simulink model "CarE_Model"  (R2019b)
settings: Solver=VariableStepAuto  StartTime=0.0  StopTime=inf  RelTol=1e-3
(part 3 of 5)

== matlab function CarE_Model/CarE_System/Mapping Module/MATLAB Function to map intensity values to facial expressions ==
  data: contribution input; anger_val output; index input; disgust_val output; fear_val output; happiness_val output; neutral_val output; sadness_val output; surprise_val output; sum output; health_factor input
function [anger_val, disgust_val, fear_val, happiness_val, neutral_val, sadness_val, surprise_val, sum] = mapping(contribution, index, health_factor)
% % we see the heaviest weightage emotion
% % we calculate face expression values for that
% % then we move to second weightage emotion
% % calculate the face expression values for that
% % so on

% health factor(hf)decides the intensity of emotion
% % FINDING NORMALIZED HF VALUE
hf = (health_factor - 3)/5;

%% INITIALIZING THE VALUES
angerexp = zeros(22,1);
disgustexp = zeros(22,1);
fearexp = zeros(22,1);
happinessexp = zeros(22,1);
neutralexp = zeros(22,1);
sadnessexp = zeros(22,1);
surpriseexp = zeros(22,1);

intensity = zeros(22,1);
%checkvalout = zeros(7,1);

% For emotion on index value 1
exp1 = index(1);
switch(exp1)
    case 1
        % joy
        happinessexp(1) = 100;
        surpriseexp(1) = 0;
        intensity(1) = 100;
    case 2 
        % distress
        sadnessexp(1) = 100;
        angerexp(1) = 0;
        intensity(1) = 100;
    case 3
        % hope
        happinessexp(1) = 100;
        surpriseexp(1) = 0;
        intensity(1) = 20;
    case 4
        % fear
        fearexp(1) = 50;
        sadnessexp(1) = 50;
        intensity(1) = 20;
    case 5
        % satisfaction
        happinessexp(1) = 100;
        surpriseexp(1) = 0;
        intensity(1) = 80;
    case 6
        % fear_confirmed
        fearexp(1) = 50;
        sadnessexp(1) = 50;
        intensity(1) = 80;
    case 7
        % relief
        happinessexp(1) = 70;
        surpriseexp(1) = 30;
        intensity(1) = 700;
    case 8
        % disappointment
        fearexp(1) = 50;
        sadnessexp(1) = 50;
        intensity(1) = 80;
    case 9
        % happy_for
        happinessexp(1) = 100;
        surpriseexp(1) = 0;
        intensity(1) = 100;
    case 10
        % sorry_for
        fearexp(1) = 50;
        sadnessexp(1) = 50;
        intensity(1) = 100;
    case 11
        % gloating
        disgustexp(1) = 50;
        happinessexp(1) = 50;
        intensity(1) = 100;
    case 12
        % resentment
        angerexp(1) = 50;
        disgustexp(1) = 50;
        intensity(1) = 100;
    case 13
        % pride
        happinessexp(1) = 100;
        surpriseexp(1) = 0;
        intensity(1) = 100;
    case 14
        % shame
        sadnessexp(1) = 50;
        angerexp(1) = 50;
        intensity(1) = 100;
    case 15
        % admiration
        happinessexp(1) = 50;
        surpriseexp(1) = 50;
        intensity(1) = 100;
    case 16
        % reproach
        angerexp(1) = 50;
        disgustexp(1) = 50;
        intensity(1) = 100;
    case 17
        % gratitude
        happinessexp(1) = 100;
        surpriseexp(1) = 0;
        intensity(1) = 100;
    case 18
        % anger
        angerexp(1) = 100;
        disgustexp(1) = 0;
        intensity(1) = 100;
    case 19
        % gratification
        happinessexp(1) = 100;
        surpriseexp(1) = 0;
        intensity(1) = 100;
    case 20
        % remorse
        sadnessexp(1) = 100;
        angerexp(1) = 0;
        intensity(1) = 100;
    case 21
        % liking
        happinessexp(1) = 70;
        surpriseexp(1) = 30;
        intensity(1) = 100;
    case 22
        % disliking
        disgustexp(1) = 100;
        happinessexp(1) = 0;
        intensity(1) = 100;
    otherwise
        neutralexp(1) = 100;
        intensity(1) = 100;
end

% For emotion on index value 2
exp2 = index(2);
switch(exp2)
    case 1
        % joy
        happinessexp(2) = 100;
        surpriseexp(2) = 0;
        intensity(2) = 100;
    case 2 
        % distress
        sadnessexp(2) = 100;
        angerexp(2) = 0;
        intensity(2) = 100;
    case 3
        % hope
        happinessexp(2) = 100;
        surpriseexp(2) = 0;
        intensity(2) = 20;
    case 4
        % fear
        fearexp(2) = 50;
        sadnessexp(2) = 50;
        intensity(2) = 20;
    case 5
        % satisfaction
        happinessexp(2) = 100;
        surpriseexp(2) = 0;
        intensity(2) = 80;
    case 6
        % fear_confirmed
        fearexp(2) = 50;
        sadnessexp(2) = 50;
        intensity(2) = 80;
    case 7
        % relief
        happinessexp(2) = 70;
        surpriseexp(2) = 30;
        intensity(2) = 700;
    case 8
        % disappointment
        fearexp(2) = 50;
        sadnessexp(2) = 50;
        intensity(2) = 80;
    case 9
        % happy_for
        happinessexp(2) = 100;
        surpriseexp(2) = 0;
        intensity(2) = 100;
    case 10
        % sorry_for
        fearexp(2) = 50;
        sadnessexp(2) = 50;
        intensity(2) = 100;
    case 11
        % gloating
        disgustexp(2) = 50;
        happinessexp(2) = 50;
        intensity(2) = 100;
    case 12
        % resentment
        angerexp(2) = 50;
        disgustexp(2) = 50;
        intensity(2) = 100;
    case 13
        % pride
        happinessexp(2) = 100;
        surpriseexp(2) = 0;
        intensity(2) = 100;
    case 14
        % shame
        sadnessexp(2) = 50;
        angerexp(2) = 50;
        intensity(2) = 100;
    case 15
        % admiration
        happinessexp(2) = 50;
        surpriseexp(2) = 50;
        intensity(2) = 100;
    case 16
        % reproach
        angerexp(2) = 50;
        disgustexp(2) = 50;
        intensity(2) = 100;
    case 17
        % gratitude
        happinessexp(2) = 100;
        surpriseexp(2) = 0;
        intensity(2) = 100;
    case 18
        % anger
        angerexp(2) = 100;
        disgustexp(2) = 0;
        intensity(2) = 100;
    case 19
        % gratification
        happinessexp(2) = 100;
        surpriseexp(2) = 0;
        intensity(2) = 100;
    case 20
        % remorse
        sadnessexp(2) = 100;
        angerexp(2) = 0;
        intensity(2) = 100;
    case 21
        % liking
        happinessexp(2) = 70;
        surpriseexp(2) = 30;
        intensity(2) = 100;
    case 22
        % disliking
        disgustexp(2) = 100;
        happinessexp(2) = 0;
        intensity(2) = 100;
    otherwise
        neutralexp(2) = 100;
        intensity(2) = 100;
end

% For emotion on index value 3
exp3 = index(3);
switch(exp3)
    case 1
        % joy
        happinessexp(3) = 100;
        surpriseexp(3) = 0;
        intensity(3) = 100;
    case 2 
        % distress
        sadnessexp(3) = 100;
        angerexp(3) = 0;
        intensity(3) = 100;
    case 3
        % hope
        happinessexp(3) = 100;
        surpriseexp(3) = 0;
        intensity(3) = 20;
    case 4
        % fear
        fearexp(3) = 50;
        sadnessexp(3) = 50;
        intensity(3) = 20;
    case 5
        % satisfaction
        happinessexp(3) = 100;
        surpriseexp(3) = 0;
        intensity(3) = 80;
    case 6
        % fear_confirmed
        fearexp(3) = 50;
        sadnessexp(3) = 50;
        intensity(3) = 80;
    case 7
        % relief
        happinessexp(3) = 70;
        surpriseexp(3) = 30;
        intensity(3) = 700;
    case 8
        % disappointment
        fearexp(3) = 50;
        sadnessexp(3) = 50;
        intensity(3) = 80;
    case 9
        % happy_for
        happinessexp(3) = 100;
        surpriseexp(3) = 0;
        intensity(3) = 100;
    case 10
        % sorry_for
        fearexp(3) = 50;
        sadnessexp(3) = 50;
        intensity(3) = 100;
    case 11
        % gloating
        disgustexp(3) = 50;
        happinessexp(3) = 50;
        intensity(3) = 100;
    case 12
        % resentment
        angerexp(3) = 50;
        disgustexp(3) = 50;
        intensity(3) = 100;
    case 13
        % pride
        happinessexp(3) = 100;
        surpriseexp(3) = 0;
        intensity(3) = 100;
    case 14
        % shame
        sadnessexp(3) = 50;
        angerexp(3) = 50;
        intensity(3) = 100;
    case 15
        % admiration
        happinessexp(3) = 50;
        surpriseexp(3) = 50;
        intensity(3) = 100;
    case 16
        % reproach
        angerexp(3) = 50;
        disgustexp(3) = 50;
        intensity(3) = 100;
    case 17
        % gratitude
        happinessexp(3) = 100;
        surpriseexp(3) = 0;
        intensity(3) = 100;
    case 18
        % anger
        angerexp(3) = 100;
        disgustexp(3) = 0;
        intensity(3) = 100;
    case 19
        % gratification
        happinessexp(3) = 100;
        surpriseexp(3) = 0;
        intensity(3) = 100;
    case 20
        % remorse
        sadnessexp(3) = 100;
        angerexp(3) = 0;
        intensity(3) = 100;
    case 21
        % liking
        happinessexp(3) = 70;
        surpriseexp(3) = 30;
        intensity(3) = 100;
    case 22
        % disliking
        disgustexp(3) = 100;
        happinessexp(3) = 0;
        intensity(3) = 100;
    otherwise
        neutralexp(3) = 100;
        intensity(3) = 100;
end

% For emotion on index value 4
exp4 = index(4);
switch(exp4)
    case 1
        % joy
        happinessexp(4) = 100;
        surpriseexp(4) = 0;
        intensity(4) = 100;
    case 2 
        % distress
        sadnessexp(4) = 100;
        angerexp(4) = 0;
        intensity(4) = 100;
    case 3
        % hope
        happinessexp(4) = 100;
        surpriseexp(4) = 0;
        intensity(4) = 20;
    case 4
        % fear
        fearexp(4) = 50;
        sadnessexp(4) = 50;
        intensity(4) = 20;
    case 5
        % satisfaction
        happinessexp(4) = 100;
        surpriseexp(4) = 0;
        intensity(4) = 80;
    case 6
        % fear_confirmed
        fearexp(4) = 50;
        sadnessexp(4) = 50;
        intensity(4) = 80;
    case 7
        % relief
        happinessexp(4) = 70;
        surpriseexp(4) = 30;
        intensity(4) = 700;
    case 8
        % disappointment
        fearexp(4) = 50;
        sadnessexp(4) = 50;
        intensity(4) = 80;
    case 9
        % happy_for
        happinessexp(4) = 100;
        surpriseexp(4) = 0;
        intensity(4) = 100;
    case 10
        % sorry_for
        fearexp(4) = 50;
        sadnessexp(4) = 50;
        intensity(4) = 100;
    case 11
        % gloating
        disgustexp(4) = 50;
        happinessexp(4) = 50;
        intensity(4) = 100;
    case 12
        % resentment
        angerexp(4) = 50;
        disgustexp(4) = 50;
        intensity(4) = 100;
    case 13
        % pride
        happinessexp(4) = 100;
        surpriseexp(4) = 0;
        intensity(4) = 100;
    case 14
        % shame
        sadnessexp(4) = 50;
        angerexp(4) = 50;
        intensity(4) = 100;
    case 15
        % admiration
        happinessexp(4) = 50;
        surpriseexp(4) = 50;
        intensity(4) = 100;
    case 16
        % reproach
        angerexp(4) = 50;
        disgustexp(4) = 50;
        intensity(4) = 100;
    case 17
        % gratitude
        happinessexp(4) = 100;
        surpriseexp(4) = 0;
        intensity(4) = 100;
    case 18
        % anger
        angerexp(4) = 100;
        disgustexp(4) = 0;
        intensity(4) = 100;
    case 19
        % gratification
        happinessexp(4) = 100;
        surpriseexp(4) = 0;
        intensity(4) = 100;
    case 20
        % remorse
        sadnessexp(4) = 100;
        angerexp(4) = 0;
        intensity(4) = 100;
    case 21
        % liking
        happinessexp(4) = 70;
        surpriseexp(4) = 30;
        intensity(4) = 100;
    case 22
        % disliking
        disgustexp(4) = 100;
        happinessexp(4) = 0;
        intensity(4) = 100;
    otherwise
        neutralexp(4) = 100;
        intensity(4) = 100;
end

% For emotion on index value 5
exp5 = index(5);
switch(exp5)
    case 1
        % joy
        happinessexp(5) = 100;
        surpriseexp(5) = 0;
        intensity(5) = 100;
    case 2 
        % distress
        sadnessexp(5) = 100;
        angerexp(5) = 0;
        intensity(5) = 100;
    case 3
        % hope
        happinessexp(5) = 100;
        surpriseexp(5) = 0;
        intensity(5) = 20;
    case 4
        % fear
        fearexp(5) = 50;
        sadnessexp(5) = 50;
        intensity(5) = 20;
    case 5
        % satisfaction
        happinessexp(5) = 100;
        surpriseexp(5) = 0;
        intensity(5) = 80;
    case 6
        % fear_confirmed
        fearexp(5) = 50;
        sadnessexp(5) = 50;
        intensity(5) = 80;
    case 7
        % relief
        happinessexp(5) = 70;
        surpriseexp(5) = 30;
        intensity(5) = 700;
    case 8
        % disappointment
        fearexp(5) = 50;
        sadnessexp(5) = 50;
        intensity(5) = 80;
    case 9
        % happy_for
        happinessexp(5) = 100;
        surpriseexp(5) = 0;
        intensity(5) = 100;
    case 10
        % sorry_for
        fearexp(5) = 50;
        sadnessexp(5) = 50;
        intensity(5) = 100;
    case 11
        % gloating
        disgustexp(5) = 50;
        happinessexp(5) = 50;
        intensity(5) = 100;
    case 12
        % resentment
        angerexp(5) = 50;
        disgustexp(5) = 50;
        intensity(5) = 100;
    case 13
        % pride
        happinessexp(5) = 100;
        surpriseexp(5) = 0;
        intensity(5) = 100;
    case 14
        % shame
        sadnessexp(5) = 50;
        angerexp(5) = 50;
        intensity(5) = 100;
    case 15
        % admiration
        happinessexp(5) = 50;
        surpriseexp(5) = 50;
        intensity(5) = 100;
    case 16
        % reproach
        angerexp(5) = 50;
        disgustexp(5) = 50;
        intensity(5) = 100;
    case 17
        % gratitude
        happinessexp(5) = 100;
        surpriseexp(5) = 0;
        intensity(5) = 100;
    case 18
        % anger
        angerexp(5) = 100;
        disgustexp(5) = 0;
        intensity(5) = 100;
    case 19
        % gratification
        happinessexp(5) = 100;
        surpriseexp(5) = 0;
        intensity(5) = 100;
    case 20
        % remorse
        sadnessexp(5) = 100;
        angerexp(5) = 0;
        intensity(5) = 100;
    case 21
        % liking
        happinessexp(5) = 70;
        surpriseexp(5) = 30;
        intensity(5) = 100;
    case 22
        % disliking
        disgustexp(5) = 100;
        happinessexp(5) = 0;
        intensity(5) = 100;
    otherwise
        neutralexp(5) = 100;
        intensity(5) = 100;
end

% For emotion on index value 6
exp6 = index(6);
switch(exp6)
    case 1
        % joy
        happinessexp(6) = 100;
        surpriseexp(6) = 0;
        intensity(6) = 100;
    case 2 
        % distress
        sadnessexp(6) = 100;
        angerexp(6) = 0;
        intensity(6) = 100;
    case 3
        % hope
        happinessexp(6) = 100;
        surpriseexp(6) = 0;
        intensity(6) = 20;
    case 4
        % fear
        fearexp(6) = 50;
        sadnessexp(6) = 50;
        intensity(6) = 20;
    case 5
        % satisfaction
        happinessexp(6) = 100;
        surpriseexp(6) = 0;
        intensity(6) = 80;
    case 6
        % fear_confirmed
        fearexp(6) = 50;
        sadnessexp(6) = 50;
        intensity(6) = 80;
    case 7
        % relief
        happinessexp(6) = 70;
        surpriseexp(6) = 30;
        intensity(6) = 700;
    case 8
        % disappointment
        fearexp(6) = 50;
        sadnessexp(6) = 50;
        intensity(6) = 80;
    case 9
        % happy_for
        happinessexp(6) = 100;
        surpriseexp(6) = 0;
        intensity(6) = 100;
    case 10
        % sorry_for
        fearexp(6) = 50;
        sadnessexp(6) = 50;
        intensity(6) = 100;
    case 11
        % gloating
        disgustexp(6) = 50;
        happinessexp(6) = 50;
        intensity(6) = 100;
    case 12
        % resentment
        angerexp(6) = 50;
        disgustexp(6) = 50;
        intensity(6) = 100;
    case 13
        % pride
        happinessexp(6) = 100;
        surpriseexp(6) = 0;
        intensity(6) = 100;
    case 14
        % shame
        sadnessexp(6) = 50;
        angerexp(6) = 50;
        intensity(6) = 100;
    case 15
        % admiration
        happinessexp(6) = 50;
        surpriseexp(6) = 50;
        intensity(6) = 100;
    case 16
        % reproach
        angerexp(6) = 50;
        disgustexp(6) = 50;
        intensity(6) = 100;
    case 17
        % gratitude
        happinessexp(6) = 100;
        surpriseexp(6) = 0;
        intensity(6) = 100;
    case 18
        % anger
        angerexp(6) = 100;
        disgustexp(6) = 0;
        intensity(6) = 100;
    case 19
        % gratification
        happinessexp(6) = 100;
        surpriseexp(6) = 0;
        intensity(6) = 100;
    case 20
        % remorse
        sadnessexp(6) = 100;
        angerexp(6) = 0;
        intensity(6) = 100;
    case 21
        % liking
        happinessexp(6) = 70;
        surpriseexp(6) = 30;
        intensity(6) = 100;
    case 22
        % disliking
        disgustexp(6) = 100;
        happinessexp(6) = 0;
        intensity(6) = 100;
    otherwise
        neutralexp(6) = 100;
        intensity(6) = 100;
end

% For emotion on index value 7
exp7 = index(7);
switch(exp7)
    case 1
        % joy
        happinessexp(7) = 100;
        surpriseexp(7) = 0;
        intensity(7) = 100;
    case 2 
        % distress
        sadnessexp(7) = 100;
        angerexp(7) = 0;
        intensity(7) = 100;
    case 3
        % hope
        happinessexp(7) = 100;
        surpriseexp(7) = 0;
        intensity(7) = 20;
    case 4
        % fear
        fearexp(7) = 50;
        sadnessexp(7) = 50;
        intensity(7) = 20;
    case 5
        % satisfaction
        happinessexp(7) = 100;
        surpriseexp(7) = 0;
        intensity(7) = 80;
    case 6
        % fear_confirmed
        fearexp(7) = 50;
        sadnessexp(7) = 50;
        intensity(7) = 80;
    case 7
        % relief
        happinessexp(7) = 70;
        surpriseexp(7) = 30;
        intensity(7) = 700;
    case 8
        % disappointment
        fearexp(7) = 50;
        sadnessexp(7) = 50;
        intensity(7) = 80;
    case 9
        % happy_for
        happinessexp(7) = 100;
        surpriseexp(7) = 0;
        intensity(7) = 100;
    case 10
        % sorry_for
        fearexp(7) = 50;
        sadnessexp(7) = 50;
        intensity(7) = 100;
    case 11
        % gloating
        disgustexp(7) = 50;
        happinessexp(7) = 50;
        intensity(7) = 100;
    case 12
        % resentment
        angerexp(7) = 50;
        disgustexp(7) = 50;
        intensity(7) = 100;
    case 13
        % pride
        happinessexp(7) = 100;
        surpriseexp(7) = 0;
        intensity(7) = 100;
    case 14
        % shame
        sadnessexp(7) = 50;
        angerexp(7) = 50;
        intensity(7) = 100;
    case 15
        % admiration
        happinessexp(7) = 50;
        surpriseexp(7) = 50;
        intensity(7) = 100;
    case 16
        % reproach
        angerexp(7) = 50;
        disgustexp(7) = 50;
        intensity(7) = 100;
    case 17
        % gratitude
        happinessexp(7) = 100;
        surpriseexp(7) = 0;
        intensity(7) = 100;
    case 18
        % anger
        angerexp(7) = 100;
        disgustexp(7) = 0;
        intensity(7) = 100;
    case 19
        % gratification
        happinessexp(7) = 100;
        surpriseexp(7) = 0;
        intensity(7) = 100;
    case 20
        % remorse
        sadnessexp(7) = 100;
        angerexp(7) = 0;
        intensity(7) = 100;
    case 21
        % liking
        happinessexp(7) = 70;
        surpriseexp(7) = 30;
        intensity(7) = 100;
    case 22
        % disliking
        disgustexp(7) = 100;
        happinessexp(7) = 0;
        intensity(7) = 100;
    otherwise
        neutralexp(7) = 100;
        intensity(7) = 100;
end

% For emotion on index value 8
exp8 = index(8);
switch(exp8)
    case 1
        % joy
        happinessexp(8) = 100;
        surpriseexp(8) = 0;
        intensity(8) = 100;
    case 2 
        % distress
        sadnessexp(8) = 100;
        angerexp(8) = 0;
        intensity(8) = 100;
    case 3
        % hope
        happinessexp(8) = 100;
        surpriseexp(8) = 0;
        intensity(8) = 20;
    case 4
        % fear
        fearexp(8) = 50;
        sadnessexp(8) = 50;
        intensity(8) = 20;
    case 5
        % satisfaction
        happinessexp(8) = 100;
        surpriseexp(8) = 0;
        intensity(8) = 80;
    case 6
        % fear_confirmed
        fearexp(8) = 50;
        sadnessexp(8) = 50;
        intensity(8) = 80;
    case 7
        % relief
        happinessexp(8) = 70;
        surpriseexp(8) = 30;
        intensity(8) = 700;
    case 8
        % disappointment
        fearexp(8) = 50;
        sadnessexp(8) = 50;
        intensity(8) = 80;
    case 9
        % happy_for
        happinessexp(8) = 100;
        surpriseexp(8) = 0;
        intensity(8) = 100;
    case 10
        % sorry_for
        fearexp(8) = 50;
        sadnessexp(8) = 50;
        intensity(8) = 100;
    case 11
        % gloating
        disgustexp(8) = 50;
        happinessexp(8) = 50;
        intensity(8) = 100;
    case 12
        % resentment
        angerexp(8) = 50;
        disgustexp(8) = 50;
        intensity(8) = 100;
    case 13
        % pride
        happinessexp(8) = 100;
        surpriseexp(8) = 0;
        intensity(8) = 100;
    case 14
        % shame
        sadnessexp(8) = 50;
        angerexp(8) = 50;
        intensity(8) = 100;
    case 15
        % admiration
        happinessexp(8) = 50;
        surpriseexp(8) = 50;
        intensity(8) = 100;
    case 16
        % reproach
        angerexp(8) = 50;
        disgustexp(8) = 50;
        intensity(8) = 100;
    case 17
        % gratitude
        happinessexp(8) = 100;
        surpriseexp(8) = 0;
        intensity(8) = 100;
    case 18
        % anger
        angerexp(8) = 100;
        disgustexp(8) = 0;
        intensity(8) = 100;
    case 19
        % gratification
        happinessexp(8) = 100;
        surpriseexp(8) = 0;
        intensity(8) = 100;
    case 20
        % remorse
        sadnessexp(8) = 100;
        angerexp(8) = 0;
        intensity(8) = 100;
    case 21
        % liking
        happinessexp(8) = 70;
        surpriseexp(8) = 30;
        intensity(8) = 100;
    case 22
        % disliking
        disgustexp(8) = 100;
        happinessexp(8) = 0;
        intensity(8) = 100;
    otherwise
        neutralexp(8) = 100;
        intensity(8) = 100;
end

% For emotion on index value 9
exp9 = index(9);
switch(exp9)
    case 1
        % joy
        happinessexp(9) = 100;
        surpriseexp(9) = 0;
        intensity(9) = 100;
    case 2 
        % distress
        sadnessexp(9) = 100;
        angerexp(9) = 0;
        intensity(9) = 100;
    case 3
        % hope
        happinessexp(9) = 100;
        surpriseexp(9) = 0;
        intensity(9) = 20;
    case 4
        % fear
        fearexp(9) = 50;
        sadnessexp(9) = 50;
        intensity(9) = 20;
    case 5
        % satisfaction
        happinessexp(9) = 100;
        surpriseexp(9) = 0;
        intensity(9) = 80;
    case 6
        % fear_confirmed
        fearexp(9) = 50;
        sadnessexp(9) = 50;
        intensity(9) = 80;
    case 7
        % relief
        happinessexp(9) = 70;
        surpriseexp(9) = 30;
        intensity(9) = 700;
    case 8
        % disappointment
        fearexp(9) = 50;
        sadnessexp(9) = 50;
        intensity(9) = 80;
    case 9
        % happy_for
        happinessexp(9) = 100;
        surpriseexp(9) = 0;
        intensity(9) = 100;
    case 10
        % sorry_for
        fearexp(9) = 50;
        sadnessexp(9) = 50;
        intensity(9) = 100;
    case 11
        % gloating
        disgustexp(9) = 50;
        happinessexp(9) = 50;
        intensity(9) = 100;
    case 12
        % resentment
        angerexp(9) = 50;
        disgustexp(9) = 50;
        intensity(9) = 100;
    case 13
        % pride
        happinessexp(9) = 100;
        surpriseexp(9) = 0;
        intensity(9) = 100;
    case 14
        % shame
        sadnessexp(9) = 50;
        angerexp(9) = 50;
        intensity(9) = 100;
    case 15
        % admiration
        happinessexp(9) = 50;
        surpriseexp(9) = 50;
        intensity(9) = 100;
    case 16
        % reproach
        angerexp(9) = 50;
        disgustexp(9) = 50;
        intensity(9) = 100;
    case 17
        % gratitude
        happinessexp(9) = 100;
        surpriseexp(9) = 0;
        intensity(9) = 100;
    case 18
        % anger
        angerexp(9) = 100;
        disgustexp(9) = 0;
        intensity(9) = 100;
    case 19
        % gratification
        happinessexp(9) = 100;
        surpriseexp(9) = 0;
        intensity(9) = 100;
    case 20
        % remorse
        sadnessexp(9) = 100;
        angerexp(9) = 0;
        intensity(9) = 100;
    case 21
        % liking
        happinessexp(9) = 70;
        surpriseexp(9) = 30;
        intensity(9) = 100;
    case 22
        % disliking
        disgustexp(9) = 100;
        happinessexp(9) = 0;
        intensity(9) = 100;
    otherwise
        neutralexp(9) = 100;
        intensity(9) = 100;
end

% For emotion on index value 10
exp10 = index(10);
switch(exp10)
    case 1
        % joy
        happinessexp(10) = 100;
        surpriseexp(10) = 0;
        intensity(10) = 100;
    case 2 
        % distress
        sadnessexp(10) = 100;
        angerexp(10) = 0;
        intensity(10) = 100;
    case 3
        % hope
        happinessexp(10) = 100;
        surpriseexp(10) = 0;
        intensity(10) = 20;
    case 4
        % fear
        fearexp(10) = 50;
        sadnessexp(10) = 50;
        intensity(10) = 20;
    case 5
        % satisfaction
        happinessexp(10) = 100;
        surpriseexp(10) = 0;
        intensity(10) = 80;
    case 6
        % fear_confirmed
        fearexp(10) = 50;
        sadnessexp(10) = 50;
        intensity(10) = 80;
    case 7
        % relief
        happinessexp(10) = 70;
        surpriseexp(10) = 30;
        intensity(10) = 700;
    case 8
        % disappointment
        fearexp(10) = 50;
        sadnessexp(10) = 50;
        intensity(10) = 80;
    case 9
        % happy_for
        happinessexp(10) = 100;
        surpriseexp(10) = 0;
        intensity(10) = 100;
    case 10
        % sorry_for
        fearexp(10) = 50;
        sadnessexp(10) = 50;
        intensity(10) = 100;
    case 11
        % gloating
        disgustexp(10) = 50;
        happinessexp(10) = 50;
        intensity(10) = 100;
    case 12
        % resentment
        angerexp(10) = 50;
        disgustexp(10) = 50;
        intensity(10) = 100;
    case 13
        % pride
        happinessexp(10) = 100;
        surpriseexp(10) = 0;
        intensity(10) = 100;
    case 14
        % shame
        sadnessexp(10) = 50;
        angerexp(10) = 50;
        intensity(10) = 100;
    case 15
        % admiration
        happinessexp(10) = 50;
        surpriseexp(10) = 50;
        intensity(10) = 100;
    case 16
        % reproach
        angerexp(10) = 50;
        disgustexp(10) = 50;
        intensity(10) = 100;
    case 17
        % gratitude
        happinessexp(10) = 100;
        surpriseexp(10) = 0;
        intensity(10) = 100;
    case 18
        % anger
        angerexp(10) = 100;
        disgustexp(10) = 0;
        intensity(10) = 100;
    case 19
        % gratification
        happinessexp(10) = 100;
        surpriseexp(10) = 0;
        intensity(10) = 100;
    case 20
        % remorse
        sadnessexp(10) = 100;
        angerexp(10) = 0;
        intensity(10) = 100;
    case 21
        % liking
        happinessexp(10) = 70;
        surpriseexp(10) = 30;
        intensity(10) = 100;
    case 22
        % disliking
        disgustexp(10) = 100;
        happinessexp(10) = 0;
        intensity(10) = 100;
    otherwise
        neutralexp(10) = 100;
        intensity(10) = 100;
end

% For emotion on index value 11
exp11 = index(11);
switch(exp11)
    case 1
        % joy
        happinessexp(11) = 100;
        surpriseexp(11) = 0;
        intensity(11) = 100;
    case 2 
        % distress
        sadnessexp(11) = 100;
        angerexp(11) = 0;
        intensity(11) = 100;
    case 3
        % hope
        happinessexp(11) = 100;
        surpriseexp(11) = 0;
        intensity(11) = 20;
    case 4
        % fear
        fearexp(11) = 50;
        sadnessexp(11) = 50;
        intensity(11) = 20;
    case 5
        % satisfaction
        happinessexp(11) = 100;
        surpriseexp(11) = 0;
        intensity(11) = 80;
    case 6
        % fear_confirmed
        fearexp(11) = 50;
        sadnessexp(11) = 50;
        intensity(11) = 80;
    case 7
        % relief
        happinessexp(11) = 70;
        surpriseexp(11) = 30;
        intensity(11) = 700;
    case 8
        % disappointment
        fearexp(11) = 50;
        sadnessexp(11) = 50;
        intensity(11) = 80;
    case 9
        % happy_for
        happinessexp(11) = 100;
        surpriseexp(11) = 0;
        intensity(11) = 100;
    case 10
        % sorry_for
        fearexp(11) = 50;
        sadnessexp(11) = 50;
        intensity(11) = 100;
    case 11
        % gloating
        disgustexp(11) = 50;
        happinessexp(11) = 50;
        intensity(11) = 100;
    case 12
        % resentment
        angerexp(11) = 50;
        disgustexp(11) = 50;
        intensity(11) = 100;
    case 13
        % pride
        happinessexp(11) = 100;
        surpriseexp(11) = 0;
        intensity(11) = 100;
    case 14
        % shame
        sadnessexp(11) = 50;
        angerexp(11) = 50;
        intensity(11) = 100;
    case 15
        % admiration
        happinessexp(11) = 50;
        surpriseexp(11) = 50;
        intensity(11) = 100;
    case 16
        % reproach
        angerexp(11) = 50;
        disgustexp(11) = 50;
        intensity(11) = 100;
    case 17
        % gratitude
        happinessexp(11) = 100;
        surpriseexp(11) = 0;
        intensity(11) = 100;
    case 18
        % anger
        angerexp(11) = 100;
        disgustexp(11) = 0;
        intensity(11) = 100;
    case 19
        % gratification
        happinessexp(11) = 100;
        surpriseexp(11) = 0;
        intensity(11) = 100;
    case 20
        % remorse
        sadnessexp(11) = 100;
        angerexp(11) = 0;
        intensity(11) = 100;
    case 21
        % liking
        happinessexp(11) = 70;
        surpriseexp(11) = 30;
        intensity(11) = 100;
    case 22
        % disliking
        disgustexp(11) = 100;
        happinessexp(11) = 0;
        intensity(11) = 100;
    otherwise
        neutralexp(11) = 100;
        intensity(11) = 100;
end

% For emotion on index value 12
exp12 = index(12);
switch(exp12)
    case 1
        % joy
        happinessexp(12) = 100;
        surpriseexp(12) = 0;
        intensity(12) = 100;
    case 2 
        % distress
        sadnessexp(12) = 100;
        angerexp(12) = 0;
        intensity(12) = 100;
    case 3
        % hope
        happinessexp(12) = 100;
        surpriseexp(12) = 0;
        intensity(12) = 20;
    case 4
        % fear
        fearexp(12) = 50;
        sadnessexp(12) = 50;
        intensity(12) = 20;
    case 5
        % satisfaction
        happinessexp(12) = 100;
        surpriseexp(12) = 0;
        intensity(12) = 80;
    case 6
        % fear_confirmed
        fearexp(12) = 50;
        sadnessexp(12) = 50;
        intensity(12) = 80;
    case 7
        % relief
        happinessexp(12) = 70;
        surpriseexp(12) = 30;
        intensity(12) = 700;
    case 8
        % disappointment
        fearexp(12) = 50;
        sadnessexp(12) = 50;
        intensity(12) = 80;
    case 9
        % happy_for
        happinessexp(12) = 100;
        surpriseexp(12) = 0;
        intensity(12) = 100;
    case 10
        % sorry_for
        fearexp(12) = 50;
        sadnessexp(12) = 50;
        intensity(12) = 100;
    case 11
        % gloating
        disgustexp(12) = 50;
        happinessexp(12) = 50;
        intensity(12) = 100;
    case 12
        % resentment
        angerexp(12) = 50;
        disgustexp(12) = 50;
        intensity(12) = 100;
    case 13
        % pride
        happinessexp(12) = 100;
        surpriseexp(12) = 0;
        intensity(12) = 100;
    case 14
        % shame
        sadnessexp(12) = 50;
        angerexp(12) = 50;
        intensity(12) = 100;
    case 15
        % admiration
        happinessexp(12) = 50;
        surpriseexp(12) = 50;
        intensity(12) = 100;
    case 16
        % reproach
        angerexp(12) = 50;
        disgustexp(12) = 50;
        intensity(12) = 100;
    case 17
        % gratitude
        happinessexp(12) = 100;
        surpriseexp(12) = 0;
        intensity(12) = 100;
    case 18
        % anger
        angerexp(12) = 100;
        disgustexp(12) = 0;
        intensity(12) = 100;
    case 19
        % gratification
        happinessexp(12) = 100;
        surpriseexp(12) = 0;
        intensity(12) = 100;
    case 20
        % remorse
        sadnessexp(12) = 100;
        angerexp(12) = 0;
        intensity(12) = 100;
    case 21
        % liking
        happinessexp(12) = 70;
        surpriseexp(12) = 30;
        intensity(12) = 100;
    case 22
        % disliking
        disgustexp(12) = 100;
        happinessexp(12) = 0;
        intensity(12) = 100;
    otherwise
        neutralexp(12) = 100;
        intensity(12) = 100;
end

% For emotion on index value 13
exp13 = index(13);
switch(exp13)
    case 1
        % joy
        happinessexp(13) = 100;
        surpriseexp(13) = 0;
        intensity(13) = 100;
    case 2 
        % distress
        sadnessexp(13) = 100;
        angerexp(13) = 0;
        intensity(13) = 100;
    case 3
        % hope
        happinessexp(13) = 100;
        surpriseexp(13) = 0;
        intensity(13) = 20;
    case 4
        % fear
        fearexp(13) = 50;
        sadnessexp(13) = 50;
        intensity(13) = 20;
    case 5
        % satisfaction
        happinessexp(13) = 100;
        surpriseexp(13) = 0;
        intensity(13) = 80;
    case 6
        % fear_confirmed
        fearexp(13) = 50;
        sadnessexp(13) = 50;
        intensity(13) = 80;
    case 7
        % relief
        happinessexp(13) = 70;
        surpriseexp(13) = 30;
        intensity(13) = 700;
    case 8
        % disappointment
        fearexp(13) = 50;
        sadnessexp(13) = 50;
        intensity(13) = 80;
    case 9
        % happy_for
        happinessexp(13) = 100;
        surpriseexp(13) = 0;
        intensity(13) = 100;
    case 10
        % sorry_for
        fearexp(13) = 50;
        sadnessexp(13) = 50;
        intensity(13) = 100;
    case 11
        % gloating
        disgustexp(13) = 50;
        happinessexp(13) = 50;
        intensity(13) = 100;
    case 12
        % resentment
        angerexp(13) = 50;
        disgustexp(13) = 50;
        intensity(13) = 100;
    case 13
        % pride
        happinessexp(13) = 100;
        surpriseexp(13) = 0;
        intensity(13) = 100;
    case 14
        % shame
        sadnessexp(13) = 50;
        angerexp(13) = 50;
        intensity(13) = 100;
    case 15
        % admiration
        happinessexp(13) = 50;
        surpriseexp(13) = 50;
        intensity(13) = 100;
    case 16
        % reproach
        angerexp(13) = 50;
        disgustexp(13) = 50;
        intensity(13) = 100;
    case 17
        % gratitude
        happinessexp(13) = 100;
        surpriseexp(13) = 0;
        intensity(13) = 100;
    case 18
        % anger
        angerexp(13) = 100;
        disgustexp(13) = 0;
        intensity(13) = 100;
    case 19
        % gratification
        happinessexp(13) = 100;
        surpriseexp(13) = 0;
        intensity(13) = 100;
    case 20
        % remorse
        sadnessexp(13) = 100;
        angerexp(13) = 0;
        intensity(13) = 100;
    case 21
        % liking
        happinessexp(13) = 70;
        surpriseexp(13) = 30;
        intensity(13) = 100;
    case 22
        % disliking
        disgustexp(13) = 100;
        happinessexp(13) = 0;
        intensity(13) = 100;
    otherwise
        neutralexp(13) = 100;
        intensity(13) = 100;
end

% For emotion on index value 14
exp14 = index(14);
switch(exp14)
    case 1
        % joy
        happinessexp(14) = 100;
        surpriseexp(14) = 0;
        intensity(14) = 100;
    case 2 
        % distress
        sadnessexp(14) = 100;
        angerexp(14) = 0;
        intensity(14) = 100;
    case 3
        % hope
        happinessexp(14) = 100;
        surpriseexp(14) = 0;
        intensity(14) = 20;
    case 4
        % fear
        fearexp(14) = 50;
        sadnessexp(14) = 50;
        intensity(14) = 20;
    case 5
        % satisfaction
        happinessexp(14) = 100;
        surpriseexp(14) = 0;
        intensity(14) = 80;
    case 6
        % fear_confirmed
        fearexp(14) = 50;
        sadnessexp(14) = 50;
        intensity(14) = 80;
    case 7
        % relief
        happinessexp(14) = 70;
        surpriseexp(14) = 30;
        intensity(14) = 700;
    case 8
        % disappointment
        fearexp(14) = 50;
        sadnessexp(14) = 50;
        intensity(14) = 80;
    case 9
        % happy_for
        happinessexp(14) = 100;
        surpriseexp(14) = 0;
        intensity(14) = 100;
    case 10
        % sorry_for
        fearexp(14) = 50;
        sadnessexp(14) = 50;
        intensity(14) = 100;
    case 11
        % gloating
        disgustexp(14) = 50;
        happinessexp(14) = 50;
        intensity(14) = 100;
    case 12
        % resentment
        angerexp(14) = 50;
        disgustexp(14) = 50;
        intensity(14) = 100;
    case 13
        % pride
        happinessexp(14) = 100;
        surpriseexp(14) = 0;
        intensity(14) = 100;
    case 14
        % shame
        sadnessexp(14) = 50;
        angerexp(14) = 50;
        intensity(14) = 100;
    case 15
        % admiration
        happinessexp(14) = 50;
        surpriseexp(14) = 50;
        intensity(14) = 100;
    case 16
        % reproach
        angerexp(14) = 50;
        disgustexp(14) = 50;
        intensity(14) = 100;
    case 17
        % gratitude
        happinessexp(14) = 100;
        surpriseexp(14) = 0;
        intensity(14) = 100;
    case 18
        % anger
        angerexp(14) = 100;
        disgustexp(14) = 0;
        intensity(14) = 100;
    case 19
        % gratification
        happinessexp(14) = 100;
        surpriseexp(14) = 0;
        intensity(14) = 100;
    case 20
        % remorse
        sadnessexp(14) = 100;
        angerexp(14) = 0;
        intensity(14) = 100;
    case 21
        % liking
        happinessexp(14) = 70;
        surpriseexp(14) = 30;
        intensity(14) = 100;
    case 22
        % disliking
        disgustexp(14) = 100;
        happinessexp(14) = 0;
        intensity(14) = 100;
    otherwise
        neutralexp(14) = 100;
        intensity(14) = 100;
end

% For emotion on index value 15
exp15 = index(15);
switch(exp15)
    case 1
        % joy
        happinessexp(15) = 100;
        surpriseexp(15) = 0;
        intensity(15) = 100;
    case 2 
        % distress
        sadnessexp(15) = 100;
        angerexp(15) = 0;
        intensity(15) = 100;
    case 3
        % hope
        happinessexp(15) = 100;
        surpriseexp(15) = 0;
        intensity(15) = 20;
    case 4
        % fear
        fearexp(15) = 50;
        sadnessexp(15) = 50;
        intensity(15) = 20;
    case 5
        % satisfaction
        happinessexp(15) = 100;
        surpriseexp(15) = 0;
        intensity(15) = 80;
    case 6
        % fear_confirmed
        fearexp(15) = 50;
        sadnessexp(15) = 50;
        intensity(15) = 80;
    case 7
        % relief
        happinessexp(15) = 70;
        surpriseexp(15) = 30;
        intensity(15) = 700;
    case 8
        % disappointment
        fearexp(15) = 50;
        sadnessexp(15) = 50;
        intensity(15) = 80;
    case 9
        % happy_for
        happinessexp(15) = 100;
        surpriseexp(15) = 0;
        intensity(15) = 100;
    case 10
        % sorry_for
        fearexp(15) = 50;
        sadnessexp(15) = 50;
        intensity(15) = 100;
    case 11
        % gloating
        disgustexp(15) = 50;
        happinessexp(15) = 50;
        intensity(15) = 100;
    case 12
        % resentment
        angerexp(15) = 50;
        disgustexp(15) = 50;
        intensity(15) = 100;
    case 13
        % pride
        happinessexp(15) = 100;
        surpriseexp(15) = 0;
        intensity(15) = 100;
    case 14
        % shame
        sadnessexp(15) = 50;
        angerexp(15) = 50;
        intensity(15) = 100;
    case 15
        % admiration
        happinessexp(15) = 50;
        surpriseexp(15) = 50;
        intensity(15) = 100;
    case 16
        % reproach
        angerexp(15) = 50;
        disgustexp(15) = 50;
        intensity(15) = 100;
    case 17
        % gratitude
        happinessexp(15) = 100;
        surpriseexp(15) = 0;
        intensity(15) = 100;
    case 18
        % anger
        angerexp(15) = 100;
        disgustexp(15) = 0;
        intensity(15) = 100;
    case 19
        % gratification
        happinessexp(15) = 100;
        surpriseexp(15) = 0;
        intensity(15) = 100;
    case 20
        % remorse
        sadnessexp(15) = 100;
        angerexp(15) = 0;
        intensity(15) = 100;
    case 21
        % liking
        happinessexp(15) = 70;
        surpriseexp(15) = 30;
        intensity(15) = 100;
    case 22
        % disliking
        disgustexp(15) = 100;
        happinessexp(15) = 0;
        intensity(15) = 100;
    otherwise
        neutralexp(15) = 100;
        intensity(15) = 100;
end

% For emotion on index value 16
exp16 = index(16);
switch(exp16)
    case 1
        % joy
        happinessexp(16) = 100;
        surpriseexp(16) = 0;
        intensity(16) = 100;
    case 2 
        % distress
        sadnessexp(16) = 100;
        angerexp(16) = 0;
        intensity(16) = 100;
    case 3
        % hope
        happinessexp(16) = 100;
        surpriseexp(16) = 0;
        intensity(16) = 20;
    case 4
        % fear
        fearexp(16) = 50;
        sadnessexp(16) = 50;
        intensity(16) = 20;
    case 5
        % satisfaction
        happinessexp(16) = 100;
        surpriseexp(16) = 0;
        intensity(16) = 80;
    case 6
        % fear_confirmed
        fearexp(16) = 50;
        sadnessexp(16) = 50;
        intensity(16) = 80;
    case 7
        % relief
        happinessexp(16) = 70;
        surpriseexp(16) = 30;
        intensity(16) = 700;
    case 8
        % disappointment
        fearexp(16) = 50;
        sadnessexp(16) = 50;
        intensity(16) = 80;
    case 9
        % happy_for
        happinessexp(16) = 100;
        surpriseexp(16) = 0;
        intensity(16) = 100;
    case 10
        % sorry_for
        fearexp(16) = 50;
        sadnessexp(16) = 50;
        intensity(16) = 100;
    case 11
        % gloating
        disgustexp(16) = 50;
        happinessexp(16) = 50;
        intensity(16) = 100;
    case 12
        % resentment
        angerexp(16) = 50;
        disgustexp(16) = 50;
        intensity(16) = 100;
    case 13
        % pride
        happinessexp(16) = 100;
        surpriseexp(16) = 0;
        intensity(16) = 100;
    case 14
        % shame
        sadnessexp(16) = 50;
        angerexp(16) = 50;
        intensity(16) = 100;
    case 15
        % admiration
        happinessexp(16) = 50;
        surpriseexp(16) = 50;
        intensity(16) = 100;
    case 16
        % reproach
        angerexp(16) = 50;
        disgustexp(16) = 50;
        intensity(16) = 100;
    case 17
        % gratitude
        happinessexp(16) = 100;
        surpriseexp(16) = 0;
        intensity(16) = 100;
    case 18
        % anger
        angerexp(16) = 100;
        disgustexp(16) = 0;
        intensity(16) = 100;
    case 19
        % gratification
        happinessexp(16) = 100;
        surpriseexp(16) = 0;
        intensity(16) = 100;
    case 20
        % remorse
        sadnessexp(16) = 100;
        angerexp(16) = 0;
        intensity(16) = 100;
    case 21
        % liking
        happinessexp(16) = 70;
        surpriseexp(16) = 30;
        intensity(16) = 100;
    case 22
        % disliking
        disgustexp(16) = 100;
        happinessexp(16) = 0;
        intensity(16) = 100;
    otherwise
        neutralexp(16) = 100;
        intensity(16) = 100;
end

% For emotion on index value 17
exp17 = index(17);
switch(exp17)
    case 1
        % joy
        happinessexp(17) = 100;
        surpriseexp(17) = 0;
        intensity(17) = 100;
    case 2 
        % distress
        sadnessexp(17) = 100;
        angerexp(17) = 0;
        intensity(17) = 100;
    case 3
        % hope
        happinessexp(17) = 100;
        surpriseexp(17) = 0;
        intensity(17) = 20;
    case 4
        % fear
        fearexp(17) = 50;
        sadnessexp(17) = 50;
        intensity(17) = 20;
    case 5
        % satisfaction
        happinessexp(17) = 100;
        surpriseexp(17) = 0;
        intensity(17) = 80;
    case 6
        % fear_confirmed
        fearexp(17) = 50;
        sadnessexp(17) = 50;
        intensity(17) = 80;
    case 7
        % relief
        happinessexp(17) = 70;
        surpriseexp(17) = 30;
        intensity(17) = 700;
    case 8
        % disappointment
        fearexp(17) = 50;
        sadnessexp(17) = 50;
        intensity(17) = 80;
    case 9
        % happy_for
        happinessexp(17) = 100;
        surpriseexp(17) = 0;
        intensity(17) = 100;
    case 10
        % sorry_for
        fearexp(17) = 50;
        sadnessexp(17) = 50;
        intensity(17) = 100;
    case 11
        % gloating
        disgustexp(17) = 50;
        happinessexp(17) = 50;
        intensity(17) = 100;
    case 12
        % resentment
        angerexp(17) = 50;
        disgustexp(17) = 50;
        intensity(17) = 100;
    case 13
        % pride
        happinessexp(17) = 100;
        surpriseexp(17) = 0;
        intensity(17) = 100;
    case 14
        % shame
        sadnessexp(17) = 50;
        angerexp(17) = 50;
        intensity(17) = 100;
    case 15
        % admiration
        happinessexp(17) = 50;
        surpriseexp(17) = 50;
        intensity(17) = 100;
    case 16
        % reproach
        angerexp(17) = 50;
        disgustexp(17) = 50;
        intensity(17) = 100;
    case 17
        % gratitude
        happinessexp(17) = 100;
        surpriseexp(17) = 0;
        intensity(17) = 100;
    case 18
        % anger
        angerexp(17) = 100;
        disgustexp(17) = 0;
        intensity(17) = 100;
    case 19
        % gratification
        happinessexp(17) = 100;
        surpriseexp(17) = 0;
        intensity(17) = 100;
    case 20
        % remorse
        sadnessexp(17) = 100;
        angerexp(17) = 0;
        intensity(17) = 100;
    case 21
        % liking
        happinessexp(17) = 70;
        surpriseexp(17) = 30;
        intensity(17) = 100;
    case 22
        % disliking
        disgustexp(17) = 100;
        happinessexp(17) = 0;
        intensity(17) = 100;
    otherwise
        neutralexp(17) = 100;
        intensity(17) = 100;
end

% For emotion on index value 18
exp18 = index(18);
switch(exp18)
    case 1
        % joy
        happinessexp(18) = 100;
        surpriseexp(18) = 0;
        intensity(18) = 100;
    case 2 
        % distress
        sadnessexp(18) = 100;
        angerexp(18) = 0;
        intensity(18) = 100;
    case 3
        % hope
        happinessexp(18) = 100;
        surpriseexp(18) = 0;
        intensity(18) = 20;
    case 4
        % fear
        fearexp(18) = 50;
        sadnessexp(18) = 50;
        intensity(18) = 20;
    case 5
        % satisfaction
        happinessexp(18) = 100;
        surpriseexp(18) = 0;
        intensity(18) = 80;
    case 6
        % fear_confirmed
        fearexp(18) = 50;
        sadnessexp(18) = 50;
        intensity(18) = 80;
    case 7
        % relief
        happinessexp(18) = 70;
        surpriseexp(18) = 30;
        intensity(18) = 700;
    case 8
        % disappointment
        fearexp(18) = 50;
        sadnessexp(18) = 50;
        intensity(18) = 80;
    case 9
        % happy_for
        happinessexp(18) = 100;
        surpriseexp(18) = 0;
        intensity(18) = 100;
    case 10
        % sorry_for
        fearexp(18) = 50;
        sadnessexp(18) = 50;
        intensity(18) = 100;
    case 11
        % gloating
        disgustexp(18) = 50;
        happinessexp(18) = 50;
        intensity(18) = 100;
    case 12
        % resentment
        angerexp(18) = 50;
        disgustexp(18) = 50;
        intensity(18) = 100;
    case 13
        % pride
        happinessexp(18) = 100;
        surpriseexp(18) = 0;
        intensity(18) = 100;
    case 14
        % shame
        sadnessexp(18) = 50;
        angerexp(18) = 50;
        intensity(18) = 100;
    case 15
        % admiration
        happinessexp(18) = 50;
        surpriseexp(18) = 50;
        intensity(18) = 100;
    case 16
        % reproach
        angerexp(18) = 50;
        disgustexp(18) = 50;
        intensity(18) = 100;
    case 17
        % gratitude
        happinessexp(18) = 100;
        surpriseexp(18) = 0;
        intensity(18) = 100;
    case 18
        % anger
        angerexp(18) = 100;
        disgustexp(18) = 0;
        intensity(18) = 100;
    case 19
        % gratification
        happinessexp(18) = 100;
        surpriseexp(18) = 0;
        intensity(18) = 100;
    case 20
        % remorse
        sadnessexp(18) = 100;
        angerexp(18) = 0;
        intensity(18) = 100;
    case 21
        % liking
        happinessexp(18) = 70;
        surpriseexp(18) = 30;
        intensity(18) = 100;
    case 22
        % disliking
        disgustexp(18) = 100;
        happinessexp(18) = 0;
        intensity(18) = 100;
    otherwise
        neutralexp(18) = 100;
        intensity(18) = 100;
end

% For emotion on index value 19
exp19 = index(19);
switch(exp19)
    case 1
        % joy
        happinessexp(19) = 100;
        surpriseexp(19) = 0;
        intensity(19) = 100;
    case 2 
        % distress
        sadnessexp(19) = 100;
        angerexp(19) = 0;
        intensity(19) = 100;
    case 3
        % hope
        happinessexp(19) = 100;
        surpriseexp(19) = 0;
        intensity(19) = 20;
    case 4
        % fear
        fearexp(19) = 50;
        sadnessexp(19) = 50;
        intensity(19) = 20;
    case 5
        % satisfaction
        happinessexp(19) = 100;
        surpriseexp(19) = 0;
        intensity(19) = 80;
    case 6
        % fear_confirmed
        fearexp(19) = 50;
        sadnessexp(19) = 50;
        intensity(19) = 80;
    case 7
        % relief
        happinessexp(19) = 70;
        surpriseexp(19) = 30;
        intensity(19) = 700;
    case 8
        % disappointment
        fearexp(19) = 50;
        sadnessexp(19) = 50;
        intensity(19) = 80;
    case 9
        % happy_for
        happinessexp(19) = 100;
        surpriseexp(19) = 0;
        intensity(19) = 100;
    case 10
        % sorry_for
        fearexp(19) = 50;
        sadnessexp(19) = 50;
        intensity(19) = 100;
    case 11
        % gloating
        disgustexp(19) = 50;
        happinessexp(19) = 50;
        intensity(19) = 100;
    case 12
        % resentment
        angerexp(19) = 50;
        disgustexp(19) = 50;
        intensity(19) = 100;
    case 13
        % pride
        happinessexp(19) = 100;
        surpriseexp(19) = 0;
        intensity(19) = 100;
    case 14
        % shame
        sadnessexp(19) = 50;
        angerexp(19) = 50;
        intensity(19) = 100;
    case 15
        % admiration
        happinessexp(19) = 50;
        surpriseexp(19) = 50;
        intensity(19) = 100;
    case 16
        % reproach
        angerexp(19) = 50;
        disgustexp(19) = 50;
        intensity(19) = 100;
    case 17
        % gratitude
        happinessexp(19) = 100;
        surpriseexp(19) = 0;
        intensity(19) = 100;
    case 18
        % anger
        angerexp(19) = 100;
        disgustexp(19) = 0;
        intensity(19) = 100;
    case 19
        % gratification
        happinessexp(19) = 100;
        surpriseexp(19) = 0;
        intensity(19) = 100;
    case 20
        % remorse
        sadnessexp(19) = 100;
        angerexp(19) = 0;
        intensity(19) = 100;
    case 21
        % liking
        happinessexp(19) = 70;
        surpriseexp(19) = 30;
        intensity(19) = 100;
    case 22
        % disliking
        disgustexp(19) = 100;
        happinessexp(19) = 0;
        intensity(19) = 100;
    otherwise
        neutralexp(19) = 100;
        intensity(19) = 100;
end

% For emotion on index value 20
exp20 = index(20);
switch(exp20)
    case 1
        % joy
        happinessexp(20) = 100;
        surpriseexp(20) = 0;
        intensity(20) = 100;
    case 2 
        % distress
        sadnessexp(20) = 100;
        angerexp(20) = 0;
        intensity(20) = 100;
    case 3
        % hope
        happinessexp(20) = 100;
        surpriseexp(20) = 0;
        intensity(20) = 20;
    case 4
        % fear
        fearexp(20) = 50;
        sadnessexp(20) = 50;
        intensity(20) = 20;
    case 5
        % satisfaction
        happinessexp(20) = 100;
        surpriseexp(20) = 0;
        intensity(20) = 80;
    case 6
        % fear_confirmed
        fearexp(20) = 50;
        sadnessexp(20) = 50;
        intensity(20) = 80;
    case 7
        % relief
        happinessexp(20) = 70;
        surpriseexp(20) = 30;
        intensity(20) = 700;
    case 8
        % disappointment
        fearexp(20) = 50;
        sadnessexp(20) = 50;
        intensity(20) = 80;
    case 9
        % happy_for
        happinessexp(20) = 100;
        surpriseexp(20) = 0;
        intensity(20) = 100;
    case 10
        % sorry_for
        fearexp(20) = 50;
        sadnessexp(20) = 50;
        intensity(20) = 100;
    case 11
        % gloating
        disgustexp(20) = 50;
        happinessexp(20) = 50;
        intensity(20) = 100;
    case 12
        % resentment
        angerexp(20) = 50;
        disgustexp(20) = 50;
        intensity(20) = 100;
    case 13
        % pride
        happinessexp(20) = 100;
        surpriseexp(20) = 0;
        intensity(20) = 100;
    case 14
        % shame
        sadnessexp(20) = 50;
        angerexp(20) = 50;
        intensity(20) = 100;
    case 15
        % admiration
        happinessexp(20) = 50;
        surpriseexp(20) = 50;
        intensity(20) = 100;
    case 16
        % reproach
        angerexp(20) = 50;
        disgustexp(20) = 50;
        intensity(20) = 100;
    case 17
        % gratitude
        happinessexp(20) = 100;
        surpriseexp(20) = 0;
        intensity(20) = 100;
    case 18
        % anger
        angerexp(20) = 100;
        disgustexp(20) = 0;
        intensity(20) = 100;
    case 19
        % gratification
        happinessexp(20) = 100;
        surpriseexp(20) = 0;
        intensity(20) = 100;
    case 20
        % remorse
        sadnessexp(20) = 100;
        angerexp(20) = 0;
        intensity(20) = 100;
    case 21
        % liking
        happinessexp(20) = 70;
        surpriseexp(20) = 30;
        intensity(20) = 100;
    case 22
        % disliking
        disgustexp(20) = 100;
        happinessexp(20) = 0;
        intensity(20) = 100;
    otherwise
        neutralexp(20) = 100;
        intensity(20) = 100;
end

% For emotion on index value 21
exp21 = index(21);
switch(exp21)
    case 1
        % joy
        happinessexp(21) = 100;
        surpriseexp(21) = 0;
        intensity(21) = 100;
    case 2 
        % distress
        sadnessexp(21) = 100;
        angerexp(21) = 0;
        intensity(21) = 100;
    case 3
        % hope
        happinessexp(21) = 100;
        surpriseexp(21) = 0;
        intensity(21) = 20;
    case 4
        % fear
        fearexp(21) = 50;
        sadnessexp(21) = 50;
        intensity(21) = 20;
    case 5
        % satisfaction
        happinessexp(21) = 100;
        surpriseexp(21) = 0;
        intensity(21) = 80;
    case 6
        % fear_confirmed
        fearexp(21) = 50;
        sadnessexp(21) = 50;
        intensity(21) = 80;
    case 7
        % relief
        happinessexp(21) = 70;
        surpriseexp(21) = 30;
        intensity(21) = 700;
    case 8
        % disappointment
        fearexp(21) = 50;
        sadnessexp(21) = 50;
        intensity(21) = 80;
    case 9
        % happy_for
        happinessexp(21) = 100;
        surpriseexp(21) = 0;
        intensity(21) = 100;
    case 10
        % sorry_for
        fearexp(21) = 50;
        sadnessexp(21) = 50;
        intensity(21) = 100;
    case 11
        % gloating
        disgustexp(21) = 50;
        happinessexp(21) = 50;
        intensity(21) = 100;
    case 12
        % resentment
        angerexp(21) = 50;
        disgustexp(21) = 50;
        intensity(21) = 100;
    case 13
        % pride
        happinessexp(21) = 100;
        surpriseexp(21) = 0;
        intensity(21) = 100;
    case 14
        % shame
        sadnessexp(21) = 50;
        angerexp(21) = 50;
        intensity(21) = 100;
    case 15
        % admiration
        happinessexp(21) = 50;
        surpriseexp(21) = 50;
        intensity(21) = 100;
    case 16
        % reproach
        angerexp(21) = 50;
        disgustexp(21) = 50;
        intensity(21) = 100;
    case 17
        % gratitude
        happinessexp(21) = 100;
        surpriseexp(21) = 0;
        intensity(21) = 100;
    case 18
        % anger
        angerexp(21) = 100;
        disgustexp(21) = 0;
        intensity(21) = 100;
    case 19
        % gratification
        happinessexp(21) = 100;
        surpriseexp(21) = 0;
        intensity(21) = 100;
    case 20
        % remorse
        sadnessexp(21) = 100;
        angerexp(21) = 0;
        intensity(21) = 100;
    case 21
        % liking
        happinessexp(21) = 70;
        surpriseexp(21) = 30;
        intensity(21) = 100;
    case 22
        % disliking
        disgustexp(21) = 100;
        happinessexp(21) = 0;
        intensity(21) = 100;
    otherwise
        neutralexp(21) = 100;
        intensity(21) = 100;
end

% For emotion on index value 22
exp22 = index(22);
switch(exp22)
    case 1
        % joy
        happinessexp(22) = 100;
        surpriseexp(22) = 0;
        intensity(22) = 100;
    case 2 
        % distress
        sadnessexp(22) = 100;
        angerexp(22) = 0;
        intensity(22) = 100;
    case 3
        % hope
        happinessexp(22) = 100;
        surpriseexp(22) = 0;
        intensity(22) = 20;
    case 4
        % fear
        fearexp(22) = 50;
        sadnessexp(22) = 50;
        intensity(22) = 20;
    case 5
        % satisfaction
        happinessexp(22) = 100;
        surpriseexp(22) = 0;
        intensity(22) = 80;
    case 6
        % fear_confirmed
        fearexp(22) = 50;
        sadnessexp(22) = 50;
        intensity(22) = 80;
    case 7
        % relief
        happinessexp(22) = 70;
        surpriseexp(22) = 30;
        intensity(22) = 700;
    case 8
        % disappointment
        fearexp(22) = 50;
        sadnessexp(22) = 50;
        intensity(22) = 80;
    case 9
        % happy_for
        happinessexp(22) = 100;
        surpriseexp(22) = 0;
        intensity(22) = 100;
    case 10
        % sorry_for
        fearexp(22) = 50;
        sadnessexp(22) = 50;
        intensity(22) = 100;
    case 11
        % gloating
        disgustexp(22) = 50;
        happinessexp(22) = 50;
        intensity(22) = 100;
    case 12
        % resentment
        angerexp(22) = 50;
        disgustexp(22) = 50;
        intensity(22) = 100;
    case 13
        % pride
        happinessexp(22) = 100;
        surpriseexp(22) = 0;
        intensity(22) = 100;
    case 14
        % shame
        sadnessexp(22) = 50;
        angerexp(22) = 50;
        intensity(22) = 100;
    case 15
        % admiration
        happinessexp(22) = 50;
        surpriseexp(22) = 50;
        intensity(22) = 100;
    case 16
        % reproach
        angerexp(22) = 50;
        disgustexp(22) = 50;
        intensity(22) = 100;
    case 17
        % gratitude
        happinessexp(22) = 100;
        surpriseexp(22) = 0;
        intensity(22) = 100;
    case 18
        % anger
        angerexp(22) = 100;
        disgustexp(22) = 0;
        intensity(22) = 100;
    case 19
        % gratification
        happinessexp(22) = 100;
        surpriseexp(22) = 0;
        intensity(22) = 100;
    case 20
        % remorse
        sadnessexp(22) = 100;
        angerexp(22) = 0;
        intensity(22) = 100;
    case 21
        % liking
        happinessexp(22) = 70;
        surpriseexp(22) = 30;
        intensity(22) = 100;
    case 22
        % disliking
        disgustexp(22) = 100;
        happinessexp(22) = 0;
        intensity(22) = 100;
    otherwise
        neutralexp(22) = 100;
        intensity(22) = 100;
end

%% CALCULATING THE FINAL PERECENTAGE VALUES FOR FACE EXPRESSIONS
%1 value of anger
anger_val = contribution(1) * angerexp(1)/100 * intensity(1)/100 + ...
    contribution(2) * angerexp(2)/100 * intensity(2)/100 +...
    contribution(3) * angerexp(3)/100 * intensity(3)/100 +...
    contribution(4) * angerexp(4)/100 * intensity(4)/100 +...
    contribution(5) * angerexp(5)/100 * intensity(5)/100 +...
    contribution(6) * angerexp(6)/100 * intensity(6)/100 +...
    contribution(7) * angerexp(7)/100 * intensity(7)/100 +...
    contribution(8) * angerexp(8)/100 * intensity(8)/100 +...
    contribution(9) * angerexp(9)/100 * intensity(9)/100 +...
    contribution(10) * angerexp(10)/100 * intensity(10)/100 +...
    contribution(11) * angerexp(11)/100 * intensity(11)/100 +...
    contribution(12) * angerexp(12)/100 * intensity(12)/100 +...
    contribution(13) * angerexp(13)/100 * intensity(13)/100 +...
    contribution(14) * angerexp(14)/100 * intensity(14)/100 +...
    contribution(15) * angerexp(15)/100 * intensity(15)/100 +...
    contribution(16) * angerexp(16)/100 * intensity(16)/100 +...
    contribution(17) * angerexp(17)/100 * intensity(17)/100 +...
    contribution(18) * angerexp(18)/100 * intensity(18)/100 +...
    contribution(19) * angerexp(19)/100 * intensity(19)/100 +...
    contribution(20) * angerexp(20)/100 * intensity(20)/100 +...
    contribution(21) * angerexp(21)/100 * intensity(21)/100 +...
    contribution(22) * angerexp(22)/100 * intensity(22)/100;

%2 value of disgust
disgust_val = contribution(1) * disgustexp(1)/100 * intensity(1)/100 + ...
    contribution(2) * disgustexp(2)/100 * intensity(2)/100 +...
    contribution(3) * disgustexp(3)/100 * intensity(3)/100 +...
    contribution(4) * disgustexp(4)/100 * intensity(4)/100 +...
    contribution(5) * disgustexp(5)/100 * intensity(5)/100 +...
    contribution(6) * disgustexp(6)/100 * intensity(6)/100 +...
    contribution(7) * disgustexp(7)/100 * intensity(7)/100 +...
    contribution(8) * disgustexp(8)/100 * intensity(8)/100 +...
    contribution(9) * disgustexp(9)/100 * intensity(9)/100 +...
    contribution(10) * disgustexp(10)/100 * intensity(10)/100 +...
    contribution(11) * disgustexp(11)/100 * intensity(11)/100 +...
    contribution(12) * disgustexp(12)/100 * intensity(12)/100 +...
    contribution(13) * disgustexp(13)/100 * intensity(13)/100 +...
    contribution(14) * disgustexp(14)/100 * intensity(14)/100 +...
    contribution(15) * disgustexp(15)/100 * intensity(15)/100 +...
    contribution(16) * disgustexp(16)/100 * intensity(16)/100 +...
    contribution(17) * disgustexp(17)/100 * intensity(17)/100 +...
    contribution(18) * disgustexp(18)/100 * intensity(18)/100 +...
    contribution(19) * disgustexp(19)/100 * intensity(19)/100 +...
    contribution(20) * disgustexp(20)/100 * intensity(20)/100 +...
    contribution(21) * disgustexp(21)/100 * intensity(21)/100 +...
    contribution(22) * disgustexp(22)/100 * intensity(22)/100;

%3 value of fear
fear_val = contribution(1) * fearexp(1)/100 * intensity(1)/100 + ...
    contribution(2) * fearexp(2)/100 * intensity(2)/100 +...
    contribution(3) * fearexp(3)/100 * intensity(3)/100 +...
    contribution(4) * fearexp(4)/100 * intensity(4)/100 +...
    contribution(5) * fearexp(5)/100 * intensity(5)/100 +...
    contribution(6) * fearexp(6)/100 * intensity(6)/100 +...
    contribution(7) * fearexp(7)/100 * intensity(7)/100 +...
    contribution(8) * fearexp(8)/100 * intensity(8)/100 +...
    contribution(9) * fearexp(9)/100 * intensity(9)/100 +...
    contribution(10) * fearexp(10)/100 * intensity(10)/100 +...
    contribution(11) * fearexp(11)/100 * intensity(11)/100 +...
    contribution(12) * fearexp(12)/100 * intensity(12)/100 +...
    contribution(13) * fearexp(13)/100 * intensity(13)/100 +...
    contribution(14) * fearexp(14)/100 * intensity(14)/100 +...
    contribution(15) * fearexp(15)/100 * intensity(15)/100 +...
    contribution(16) * fearexp(16)/100 * intensity(16)/100 +...
    contribution(17) * fearexp(17)/100 * intensity(17)/100 +...
    contribution(18) * fearexp(18)/100 * intensity(18)/100 +...
    contribution(19) * fearexp(19)/100 * intensity(19)/100 +...
    contribution(20) * fearexp(20)/100 * intensity(20)/100 +...
    contribution(21) * fearexp(21)/100 * intensity(21)/100 +...
    contribution(22) * fearexp(22)/100 * intensity(22)/100;

%4 value of happiness
happiness_val = contribution(1) * happinessexp(1)/100 * intensity(1)/100 + ...
    contribution(2) * happinessexp(2)/100 * intensity(2)/100 +...
    contribution(3) * happinessexp(3)/100 * intensity(3)/100 +...
    contribution(4) * happinessexp(4)/100 * intensity(4)/100 +...
    contribution(5) * happinessexp(5)/100 * intensity(5)/100 +...
    contribution(6) * happinessexp(6)/100 * intensity(6)/100 +...
    contribution(7) * happinessexp(7)/100 * intensity(7)/100 +...
    contribution(8) * happinessexp(8)/100 * intensity(8)/100 +...
    contribution(9) * happinessexp(9)/100 * intensity(9)/100 +...
    contribution(10) * happinessexp(10)/100 * intensity(10)/100 +...
    contribution(11) * happinessexp(11)/100 * intensity(11)/100 +...
    contribution(12) * happinessexp(12)/100 * intensity(12)/100 +...
    contribution(13) * happinessexp(13)/100 * intensity(13)/100 +...
    contribution(14) * happinessexp(14)/100 * intensity(14)/100 +...
    contribution(15) * happinessexp(15)/100 * intensity(15)/100 +...
    contribution(16) * happinessexp(16)/100 * intensity(16)/100 +...
    contribution(17) * happinessexp(17)/100 * intensity(17)/100 +...
    contribution(18) * happinessexp(18)/100 * intensity(18)/100 +...
    contribution(19) * happinessexp(19)/100 * intensity(19)/100 +...
    contribution(20) * happinessexp(20)/100 * intensity(20)/100 +...
    contribution(21) * happinessexp(21)/100 * intensity(21)/100 +...
    contribution(22) * happinessexp(22)/100 * intensity(22)/100;

%5 value of neutral
neutral_val = contribution(1) * neutralexp(1)/100 * intensity(1)/100 + ...
    contribution(2) * neutralexp(2)/100 * intensity(2)/100 +...
    contribution(3) * neutralexp(3)/100 * intensity(3)/100 +...
    contribution(4) * neutralexp(4)/100 * intensity(4)/100 +...
    contribution(5) * neutralexp(5)/100 * intensity(5)/100 +...
    contribution(6) * neutralexp(6)/100 * intensity(6)/100 +...
    contribution(7) * neutralexp(7)/100 * intensity(7)/100 +...
    contribution(8) * neutralexp(8)/100 * intensity(8)/100 +...
    contribution(9) * neutralexp(9)/100 * intensity(9)/100 +...
    contribution(10) * neutralexp(10)/100 * intensity(10)/100 +...
    contribution(11) * neutralexp(11)/100 * intensity(11)/100 +...
    contribution(12) * neutralexp(12)/100 * intensity(12)/100 +...
    contribution(13) * neutralexp(13)/100 * intensity(13)/100 +...
    contribution(14) * neutralexp(14)/100 * intensity(14)/100 +...
    contribution(15) * neutralexp(15)/100 * intensity(15)/100 +...
    contribution(16) * neutralexp(16)/100 * intensity(16)/100 +...
    contribution(17) * neutralexp(17)/100 * intensity(17)/100 +...
    contribution(18) * neutralexp(18)/100 * intensity(18)/100 +...
    contribution(19) * neutralexp(19)/100 * intensity(19)/100 +...
    contribution(20) * neutralexp(20)/100 * intensity(20)/100 +...
    contribution(21) * neutralexp(21)/100 * intensity(21)/100 +...
    contribution(22) * neutralexp(22)/100 * intensity(22)/100;

%6 value of sadness
sadness_val = contribution(1) * sadnessexp(1)/100 * intensity(1)/100 + ...
    contribution(2) * sadnessexp(2)/100 * intensity(2)/100 +...
    contribution(3) * sadnessexp(3)/100 * intensity(3)/100 +...
    contribution(4) * sadnessexp(4)/100 * intensity(4)/100 +...
    contribution(5) * sadnessexp(5)/100 * intensity(5)/100 +...
    contribution(6) * sadnessexp(6)/100 * intensity(6)/100 +...
    contribution(7) * sadnessexp(7)/100 * intensity(7)/100 +...
    contribution(8) * sadnessexp(8)/100 * intensity(8)/100 +...
    contribution(9) * sadnessexp(9)/100 * intensity(9)/100 +...
    contribution(10) * sadnessexp(10)/100 * intensity(10)/100 +...
    contribution(11) * sadnessexp(11)/100 * intensity(11)/100 +...
    contribution(12) * sadnessexp(12)/100 * intensity(12)/100 +...
    contribution(13) * sadnessexp(13)/100 * intensity(13)/100 +...
    contribution(14) * sadnessexp(14)/100 * intensity(14)/100 +...
    contribution(15) * sadnessexp(15)/100 * intensity(15)/100 +...
    contribution(16) * sadnessexp(16)/100 * intensity(16)/100 +...
    contribution(17) * sadnessexp(17)/100 * intensity(17)/100 +...
    contribution(18) * sadnessexp(18)/100 * intensity(18)/100 +...
    contribution(19) * sadnessexp(19)/100 * intensity(19)/100 +...
    contribution(20) * sadnessexp(20)/100 * intensity(20)/100 +...
    contribution(21) * sadnessexp(21)/100 * intensity(21)/100 +...
    contribution(22) * sadnessexp(22)/100 * intensity(22)/100;

%7 value of surprise
surprise_val = contribution(1) * surpriseexp(1)/100 * intensity(1)/100 + ...
    contribution(2) * surpriseexp(2)/100 * intensity(2)/100 +...
    contribution(3) * surpriseexp(3)/100 * intensity(3)/100 +...
    contribution(4) * surpriseexp(4)/100 * intensity(4)/100 +...
    contribution(5) * surpriseexp(5)/100 * intensity(5)/100 +...
    contribution(6) * surpriseexp(6)/100 * intensity(6)/100 +...
    contribution(7) * surpriseexp(7)/100 * intensity(7)/100 +...
    contribution(8) * surpriseexp(8)/100 * intensity(8)/100 +...
    contribution(9) * surpriseexp(9)/100 * intensity(9)/100 +...
    contribution(10) * surpriseexp(10)/100 * intensity(10)/100 +...
    contribution(11) * surpriseexp(11)/100 * intensity(11)/100 +...
    contribution(12) * surpriseexp(12)/100 * intensity(12)/100 +...
    contribution(13) * surpriseexp(13)/100 * intensity(13)/100 +...
    contribution(14) * surpriseexp(14)/100 * intensity(14)/100 +...
    contribution(15) * surpriseexp(15)/100 * intensity(15)/100 +...
    contribution(16) * surpriseexp(16)/100 * intensity(16)/100 +...
    contribution(17) * surpriseexp(17)/100 * intensity(17)/100 +...
    contribution(18) * surpriseexp(18)/100 * intensity(18)/100 +...
    contribution(19) * surpriseexp(19)/100 * intensity(19)/100 +...
    contribution(20) * surpriseexp(20)/100 * intensity(20)/100 +...
    contribution(21) * surpriseexp(21)/100 * intensity(21)/100 +...
    contribution(22) * surpriseexp(22)/100 * intensity(22)/100;

%including hf in calculation
if(hf >= 0)
    anger_val = abs(anger_val * abs(hf));
    disgust_val = abs(disgust_val * abs(hf));
    fear_val = abs(fear_val * abs(hf));
    happiness_val = abs(happiness_val / abs(hf));
    sadness_val = abs(sadness_val * abs(hf));
    surprise_val = abs(surprise_val * abs(hf));
end
if(hf < 0)
    anger_val = abs(anger_val / abs(hf));
    disgust_val = abs(disgust_val / abs(hf));
    fear_val = abs(fear_val / abs(hf));
    happiness_val = abs(happiness_val * abs(hf));
    sadness_val = abs(sadness_val / abs(hf));
    surprise_val = abs(surprise_val / abs(hf));
end

sum_of_vals = anger_val + disgust_val + fear_val + happiness_val + neutral_val + sadness_val + surprise_val;
anger_val = anger_val * 1/sum_of_vals;
disgust_val = disgust_val * 1/sum_of_vals;
fear_val = fear_val * 1/sum_of_vals;
happiness_val = happiness_val * 1/sum_of_vals;
neutral_val = neutral_val * 1/sum_of_vals;
sadness_val = sadness_val * 1/sum_of_vals;
surprise_val = surprise_val * 1/sum_of_vals;
sum = anger_val + disgust_val + fear_val + happiness_val + neutral_val + sadness_val + surprise_val;
end
